simulink model "plane_model"  (R2022a)
settings: Solver=VariableStepAuto  StartTime=0.0  StopTime=0.18  RelTol=1e-3
values from neighbouring files (symbols this model uses):
  Kp = 147    [main.m]
settings Model: Creator=punk  LastModifiedBy=punk

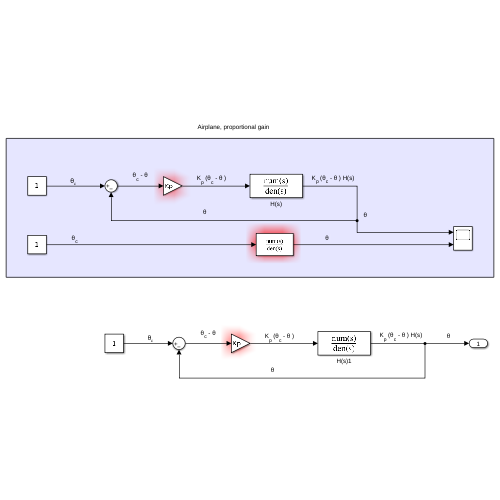
[thumbnail: Simulink's stored preview of the top-level diagram]
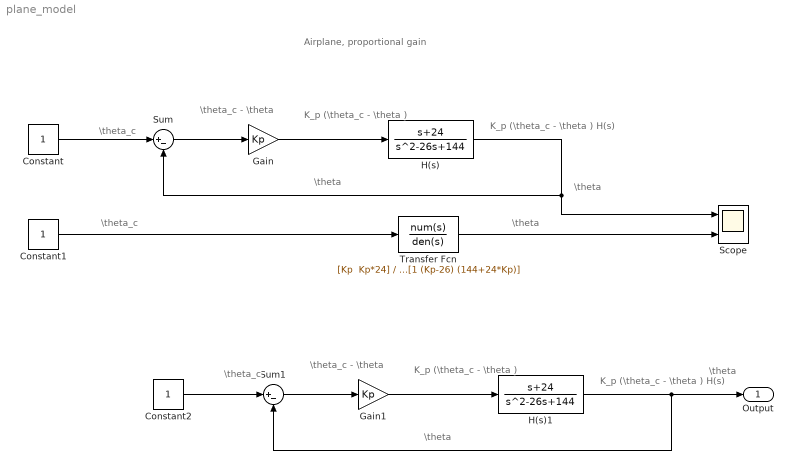
== system plane_model ==
  note: \theta_c
  note: K_p (\theta_c - \theta ) H(s)
  note: K_p (\theta_c - \theta )
  note: \theta_c - \theta
  note: Airplane, proportional gain
  note: \theta
  note: \theta_c
  note: \theta
  note: \theta
  note: \theta_c - \theta
  note: \theta_c
  note: \theta
  note: K_p (\theta_c - \theta ) H(s)
  note: K_p (\theta_c - \theta )
  note: \theta
  Constant : Constant
  Constant1 : Constant
  Constant2 : Constant
  Gain : Gain  Gain=Kp
  Gain1 : Gain  Gain=Kp
  H(s) : TransferFcn  Numerator=[1 24]  Denominator=[1 -26 144]
  H(s)1 : TransferFcn  Numerator=[1 24]  Denominator=[1 -26 144]
  Scope : Scope  NumInputPorts=2
  Sum : Sum  Inputs=|+-
  Sum1 : Sum  Inputs=|+-
  Transfer Fcn : TransferFcn  Numerator="[Kp  Kp*24]"  Denominator=[1 (Kp-26) (144+24*Kp)]
  Output : Outport
  wires:
  Gain/1 -> H(s)/1
  Sum/1 -> Gain/1
  Constant/1 -> Sum/1
  H(s)/1 -> Scope/1, Sum/2
  Constant1/1 -> Transfer Fcn/1
  Transfer Fcn/1 -> Scope/2
  Gain1/1 -> H(s)1/1
  H(s)1/1 -> Output/1, Sum1/2
  Constant2/1 -> Sum1/1
  Sum1/1 -> Gain1/1
